simulink library "EndStopChecker"  (R2016b)
settings: Solver=VariableStepAuto  StartTime=0.0  StopTime=10.0  RelTol=1e-3
libraries: EndStopChecker x4
settings Model: Creator=Marc  LastModifiedBy=march

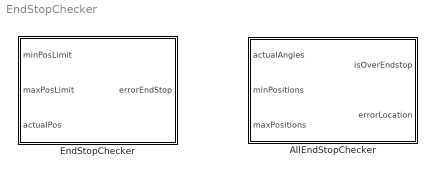
== system EndStopChecker ==
  AllEndStopChecker : Subsystem
  EndStopChecker : Subsystem

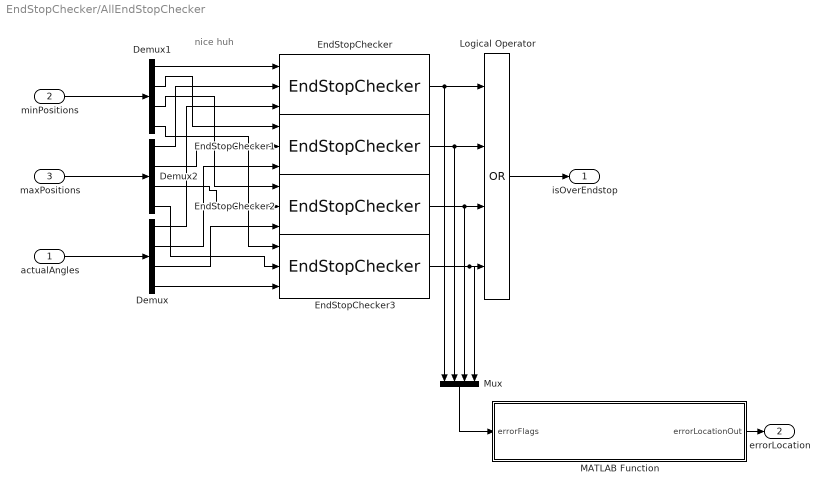
== system EndStopChecker/AllEndStopChecker ==
  note: nice huh
  actualAngles : Inport
  minPositions : Inport  Port=2
  maxPositions : Inport  Port=3
  Demux : Demux
  Demux1 : Demux
  Demux2 : Demux
  EndStopChecker{,1..3} (4 alike) : EndStopChecker/EndStopChecker
  Logical Operator : Logic  Operator=OR  Inputs=4  AllPortsSameDT=off  OutDataTypeStr=boolean
  MATLAB Function : MATLAB Function  TreatAsAtomicUnit=on
  Mux : Mux
  isOverEndstop : Outport
  errorLocation : Outport  Port=2
  wires:
  Mux/1 -> MATLAB Function/1(errorFlags)
  MATLAB Function/1(errorLocationOut) -> errorLocation/1
  actualAngles/1 -> Demux/1
  minPositions/1 -> Demux1/1
  maxPositions/1 -> Demux2/1
  Demux1/1 -> EndStopChecker/1
  Demux2/1 -> EndStopChecker/2
  Demux/1 -> EndStopChecker/3
  Demux1/2 -> EndStopChecker1/1
  Demux2/2 -> EndStopChecker1/2
  Demux/2 -> EndStopChecker1/3
  Demux1/3 -> EndStopChecker2/1
  Demux2/3 -> EndStopChecker2/2
  Demux/3 -> EndStopChecker2/3
  Demux1/4 -> EndStopChecker3/1
  Demux2/4 -> EndStopChecker3/2
  Demux/4 -> EndStopChecker3/3
  EndStopChecker1/1 -> Logical Operator/2, Mux/2
  EndStopChecker2/1 -> Logical Operator/3, Mux/3
  EndStopChecker3/1 -> Logical Operator/4, Mux/4
  EndStopChecker/1 -> Logical Operator/1, Mux/1
  Logical Operator/1 -> isOverEndstop/1

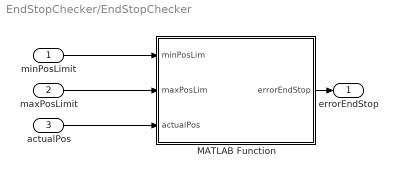
== system EndStopChecker/EndStopChecker ==
  minPosLimit : Inport
  maxPosLimit : Inport  Port=2
  actualPos : Inport  Port=3
  MATLAB Function : MATLAB Function  TreatAsAtomicUnit=on
  errorEndStop : Outport
  wires:
  minPosLimit/1 -> MATLAB Function/1(minPosLim)
  actualPos/1 -> MATLAB Function/3(actualPos)
  maxPosLimit/1 -> MATLAB Function/2(maxPosLim)
  MATLAB Function/1(errorEndStop) -> errorEndStop/1

== matlab function EndStopChecker/AllEndStopChecker/MATLAB Function ==
  data: errorFlags input; errorLocationOut output
function errorLocationOut = getErrorLocationFromErrorFlags(errorFlags)
errorLocation = '00000000';
for i=1:4
    errorLocation(i) = log2char(errorFlags(i)>0);
end
errorLocationOut = bin2dec(errorLocation);

== matlab function EndStopChecker/MATLAB Function ==
  data: minPosLim input; errorEndStop output; maxPosLim input; actualPos input
function errorEndStop = fcn(minPosLim, maxPosLim, actualPos)
%check end stops

if actualPos <= minPosLim
    errorEndStop =1;
elseif actualPos >= maxPosLim
    errorEndStop =1;
else 
    errorEndStop =0;
end
